simulink model "sim_P"  (R2019a)
settings: Solver=FixedStepAuto  StartTime=0.0  StopTime=end_time  FixedStep=FStep  RelTol=1e-3  EnableMultiTasking=on
undefined symbols (not defined in the file): d, h, k, K, T
settings Model: Creator=user  LastModifiedBy=ogure
settings SolverCC: SolverResetMethod=Robust
settings DataIOCC: LimitDataPoints=on  SaveFormat=Array  SaveOutput=off  ReturnWorkspaceOutputs=off  OutputSaveName=X,X1,X2,X3,X4,L,H
settings OptimizationCC: LifeSpan=inf
settings DebuggingCC: SolverPrmCheckMsg=warning  SFUnexpectedBacktrackingDiag=warning  SFNoUnconditionalDefaultTransitionDiag=warning  SFExecutionAtInitializationDiag=none  ArithmeticOperatorsInVariantConditions=warning
settings HardwareCC: ProdBitPerPointer=32  ProdBitPerSizeT=32  ProdBitPerPtrDiffT=32  ProdLargestAtomicFloat=None  ProdIntDivRoundTo=Undefined  ProdEndianess=Unspecified  ProdWordSize=32  ProdHWDeviceType=32-bit Generic
settings ModelReferenceCC: PropagateSignalLabelsOutOfModel=off
settings SFSimCC: SimUseLocalCustomCode=off
settings RTWCC: RTWUseLocalCustomCode=off
settings CodeAppCC: StateflowObjectComments=on
settings GRTTargetCC: TargetLangStandard=C89/C90 (ANSI)  GeneratePreprocessorConditionals=Disable all
settings ConfigComp: CovMetricSettings=dw  CovHtmlReporting=on  CovSaveCumulativeToWorkspaceVar=on  CovSaveSingleToWorkspaceVar=on  CovExternalEMLEnable=off  CovSFcnEnable=off

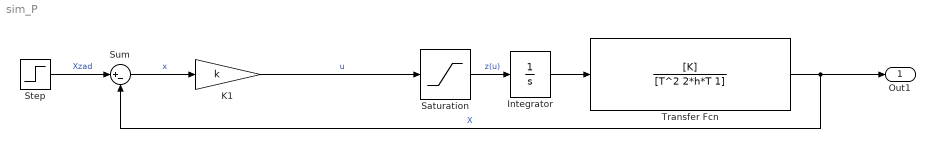
== system sim_P ==
  Integrator : Integrator
  K1 : Gain  Gain=k
  Saturation : Saturate  UpperLimit=d  LowerLimit=-d
  Step : Step  SampleTime=0
  Sum : Sum  Inputs=|+-
  Transfer Fcn : TransferFcn  Numerator=[K]  Denominator=[T^2 2*h*T 1]
  Out1 : Outport  SignalName=X
  wires:
  Transfer Fcn/1 -> Sum/2, Out1/1  "X"
  Integrator/1 -> Transfer Fcn/1
  Step/1 -> Sum/1  "Xzad"
  K1/1 -> Saturation/1  "u"
  Saturation/1 -> Integrator/1  "z(u)"
  Sum/1 -> K1/1  "x"
